simulink model "adaptive_mrac_comp_mod"  (R2020a)
settings: Solver=FixedStepAuto  StartTime=0.0  StopTime=10  FixedStep=0.01  RelTol=1e-3
values from neighbouring files (symbols this model uses):
  gamma_x = [0.5; 0.5]    [cases_test.m]    (also in cases_tests_lr.m = gamma_x_0 * i; mrac_model_const_ref.m = params(4:5); mrac_model_e2y.m = params(7:8); mrac_model_e2y_2delay.m = params(7:8))
  k_x0 = k_x0_list(:, plant_case)    [cases_test.m]    (also in mrac_model_const_ref.m = [-params(1); params(2)]; mrac_model_e2y.m = params(1:2); mrac_model_e2y_2delay.m = params(1:2); mrac_model_lr_init.m = [-params(1); params(2)])
  P = lyap(ref_sys.A', eye(2))    [cases_test.m]    (also in cases_tests_lr.m; mrac_model_e2y.m = [10, .2; 10, .2]; mrac_model_e2y_2delay.m = [1.5, 0; 1.5, 3.5]; mrac_model_lr_init_low_pass_comp.m = params(3:4))
  ref_sys = canon(ref_sys, 'modal')    [cases_test.m]    (also in cases_tests_lr.m; mrac_model.m = ss([tf_cl_pade; s*tf_cl_pade]); mrac_model_e2y.m = ss([tf_cl_pade; s*tf_cl_pade]); mrac_model_e2y_2delay.m = ss([tf_cl_pade; s*tf_cl_pade]))
undefined symbols (not defined in the file or in its folder): case_, ref_x0
settings Model: OrderedModelArguments=off  Creator=lorenzoterenzi  LastModifiedBy=lorenzoterenzi

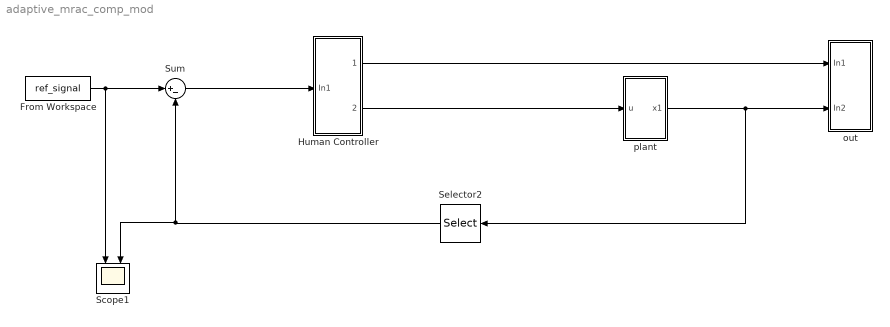
== system adaptive_mrac_comp_mod ==
  From Workspace : FromWorkspace  VariableName=ref_signal
  Human Controller : Subsystem
  Scope1 : Scope  NumInputPorts=2
  Selector2 : Selector  InputPortWidth=2  IndexOptions=Index vector (dialog)  Indices=[1]  OutputSizes=1
  Sum : Sum  Inputs=|+-
  out : Subsystem
  plant : Subsystem
  wires:
  plant/1(x1) -> out/2(In2), Selector2/1
  From Workspace/1 -> Sum/1, Scope1/1
  Selector2/1 -> Scope1/2, Sum/2
  Sum/1 -> Human Controller/1(In1)
  Human Controller/1(Out1) -> out/1(In1)
  Human Controller/2(Out2) -> plant/1(u)

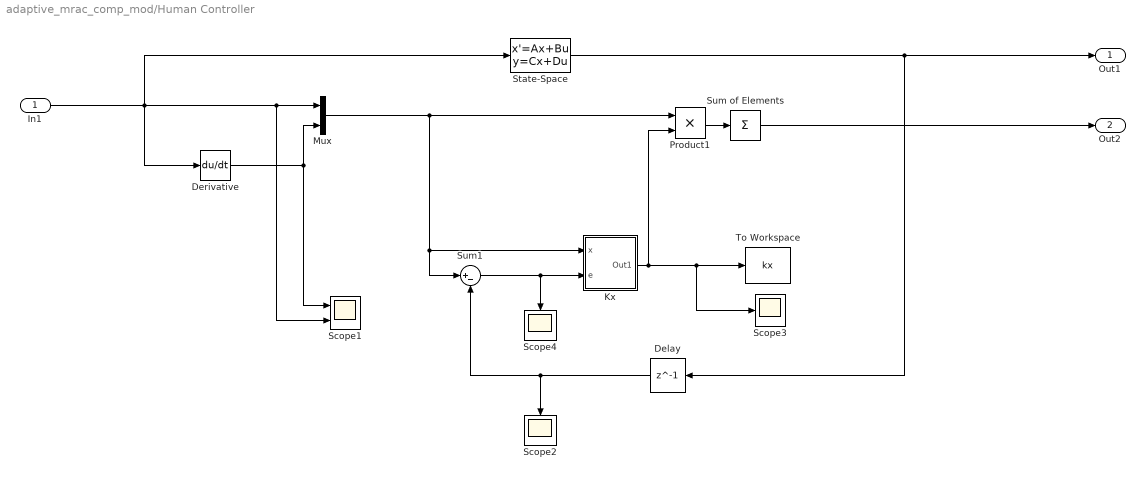
== system adaptive_mrac_comp_mod/Human Controller ==
  In1 : Inport
  Delay : Delay  DelayLength=1  InitialCondition=0
  Derivative : Derivative
  Kx : Subsystem
  Mux : Mux  Inputs=2
  Product1 : Product
  Scope1 : Scope  NumInputPorts=2
  Scope2 : Scope
  Scope3 : Scope
  Scope4 : Scope
  State-Space : StateSpace  A=ref_sys.A  B=ref_sys.B  C=ref_sys.C  D=ref_sys.D  InitialCondition=ref_x0
  Sum of Elements : Sum  Inputs=+
  Sum1 : Sum  Inputs=|+-
  To Workspace : ToWorkspace  VariableName=kx  SaveFormat=Timeseries  SampleTime=-1
  Out1 : Outport
  Out2 : Outport  Port=2
  wires:
  State-Space/1 -> Delay/1, Out1/1
  Mux/1 -> Sum1/1, Kx/1(x), Product1/1
  Sum of Elements/1 -> Out2/1
  Product1/1 -> Sum of Elements/1
  Sum1/1 -> Scope4/1, Kx/2(e)
  In1/1 -> Scope1/2, Mux/1, Derivative/1, State-Space/1
  Kx/1(Out1) -> Product1/2, Scope3/1, To Workspace/1
  Derivative/1 -> Mux/2, Scope1/1
  Delay/1 -> Sum1/2, Scope2/1

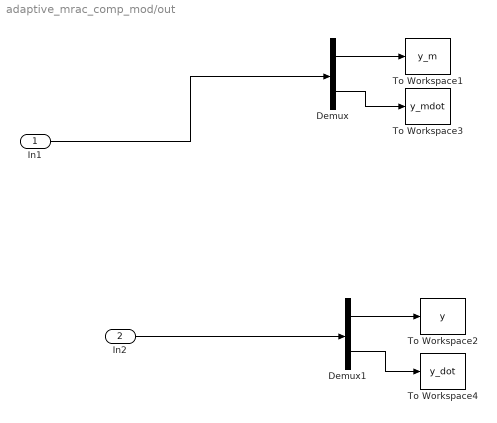
== system adaptive_mrac_comp_mod/out ==
  In1 : Inport
  In2 : Inport  Port=2
  Demux : Demux  Outputs=2
  Demux1 : Demux  Outputs=2
  To Workspace1 : ToWorkspace  VariableName=y_m  SaveFormat=Timeseries  SampleTime=-1
  To Workspace2 : ToWorkspace  VariableName=y  SaveFormat=Timeseries  SampleTime=-1
  To Workspace3 : ToWorkspace  VariableName=y_mdot  SaveFormat=Timeseries  SampleTime=-1
  To Workspace4 : ToWorkspace  VariableName=y_dot  SaveFormat=Timeseries  SampleTime=-1
  wires:
  Demux/2 -> To Workspace3/1
  Demux1/1 -> To Workspace2/1
  Demux1/2 -> To Workspace4/1
  In2/1 -> Demux1/1
  In1/1 -> Demux/1
  Demux/1 -> To Workspace1/1

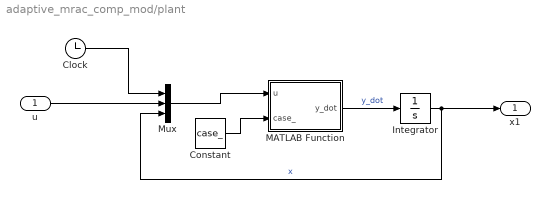
== system adaptive_mrac_comp_mod/plant ==
  u : Inport
  Clock : Clock
  Constant : Constant  Value=case_
  Integrator : Integrator  InitialCondition=[0;0]
  MATLAB Function : MATLAB Function  TreatAsAtomicUnit=on
  Mux : Mux  Inputs=3
  x1 : Outport
  wires:
  Mux/1 -> MATLAB Function/1(u)
  Integrator/1 -> x1/1, Mux/3  "x"
  MATLAB Function/1(y_dot) -> Integrator/1  "y_dot"
  Clock/1 -> Mux/1
  Constant/1 -> MATLAB Function/2(case_)
  u/1 -> Mux/2

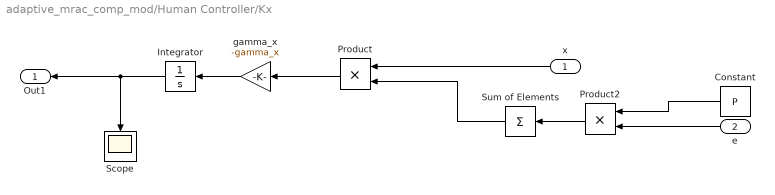
== system adaptive_mrac_comp_mod/Human Controller/Kx ==
  x : Inport
  e : Inport  Port=2
  Constant : Constant  Value=P
  Integrator : Integrator  InitialCondition=k_x0
  Product : Product
  Product2 : Product
  Scope : Scope
  Sum of Elements : Sum  Inputs=+
  gamma_x : Gain  Gain=-gamma_x
  Out1 : Outport  PortDimensions=[2, 1]
  wires:
  x/1 -> Product/1
  e/1 -> Product2/2
  Product2/1 -> Sum of Elements/1
  Sum of Elements/1 -> Product/2
  Integrator/1 -> Out1/1, Scope/1
  Constant/1 -> Product2/1
  gamma_x/1 -> Integrator/1
  Product/1 -> gamma_x/1

== matlab function adaptive_mrac_comp_mod/plant/MATLAB Function ==
  data: u input size=4; y_dot output size=2; case_ input
function y_dot = fcn(u, case_)
    t = u(1);
    u_c = u(2);
    y_prev = u(3:4);
    y_dot = models.peter_plant(case_, t, u_c, y_prev);
end


% function y_dot = peter_plant(case_, t, u, y_prev)
%     % case 1: first to second order system transition
%     if case_ == 1
%         M = -1;
%         G = -100;
%     % case 2: second to first order transition
%     elseif case_ == 2 
%         M = 91;
%         G = 100;
%     elseif case_ == 3    
%         M = 50;
%         G = 0.5;
%     elseif case_ == 4
%         M = 50;
%         G = 100;
%     else
%         G = 0;
%         M = 0;
%     end
% 
%     omega_b1 = 6;
%     omega_b2 = 0.2;
%     k_c1 = 90;
%     k_c2 = 30;
% 
%     omega_b = omega_b1 + (omega_b2 - omega_b1)./(1 + exp(-G * (t - M)));
%     k_c = k_c1 + (k_c2 - k_c1)./(1 + exp(-G * (t - M)));
% 
%     A = [0, 1; 0, omega_b];
%     B = [0; k_c];
%     y_dot = A*y_prev + B*u;
% end
